simulink model "EvenorOddcheck"  (R2021a)
settings: Solver=FixedStepDiscrete  StartTime=0.0  StopTime=10.0  RelTol=1e-3
libraries: simulink x1
settings Model: Creator=Dell  LastModifiedBy=Dell
settings OptimizationCC: DefaultParameterBehavior=Inlined  EnhancedBackFolding=on  PassReuseOutputArgsAs=Individual arguments  ZeroExternalMemoryAtStartup=off  ZeroInternalMemoryAtStartup=off  OptimizeBlockOrder=speed  DifferentSizesBufferReuse=on  OptimizationCustomize=off  EfficientTunableParamExpr=on
settings DebuggingCC: ParameterTunabilityLossMsg=error
settings SFSimCC: MATLABDynamicMemAlloc=off
settings RTWCC: SystemTargetFile=ert.tlc  GenCodeOnly=on  TemplateMakefile=ert_default_tmf  GenerateReport=on  IncludeHyperlinkInReport=on  LaunchReport=on  GenerateTraceInfo=on
settings CodeAppCC: ForceParamTrailComments=on  IgnoreCustomStorageClasses=off  OperatorAnnotations=on  SimulinkDataObjDesc=on  SFDataObjDesc=on  InsertBlockDesc=on
settings ERTTargetCC: TargetLangStandard=C99 (ISO)  GenerateSampleERTMain=on  InlinedParameterPlacement=NonHierarchical  ERTCustomFileTemplate=example_file_process.tlc

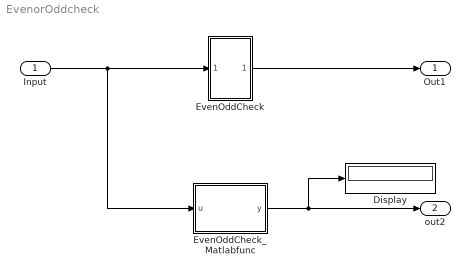
== system EvenorOddcheck ==
  Input : Inport  OutDataTypeStr=uint8
  Display : Display
  EvenOddCheck : Subsystem
  EvenOddCheck_Matlabfunc : MATLAB Function  TreatAsAtomicUnit=on
  Out1 : Outport  OutDataTypeStr=string
  out2 : Outport  Port=2
  wires:
  Input/1 -> EvenOddCheck_Matlabfunc/1(u), EvenOddCheck/1(In1)
  EvenOddCheck/1(Out1) -> Out1/1
  EvenOddCheck_Matlabfunc/1(y) -> Display/1, out2/1

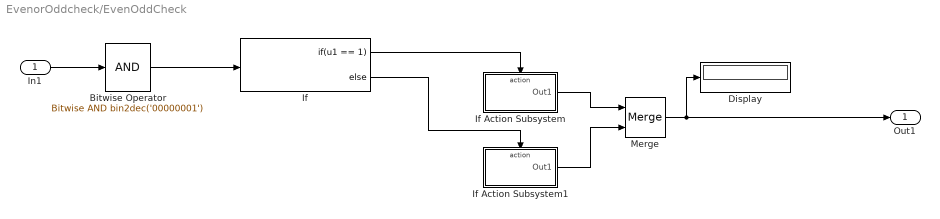
== system EvenorOddcheck/EvenOddCheck ==
  In1 : Inport
  Bitwise Operator : simulink/Logic and Bit Operations/Bitwise Operator  logicop=AND  UseBitMask=on  BitMask=bin2dec('00000001')  BitMaskRealWorld=Stored Integer
  Display : Display
  If : If  IfExpression=u1 == 1
  If Action Subsystem : Subsystem  TreatAsAtomicUnit=on
  If Action Subsystem1 : Subsystem  TreatAsAtomicUnit=on
  Merge : Merge
  Out1 : Outport
  wires:
  Bitwise Operator/1 -> If/1
  If Action Subsystem/1(Out1) -> Merge/1
  If Action Subsystem1/1(Out1) -> Merge/2
  In1/1 -> Bitwise Operator/1
  If/2 -> If Action Subsystem1/Action
  Merge/1 -> Out1/1, Display/1
  If/1 -> If Action Subsystem/Action

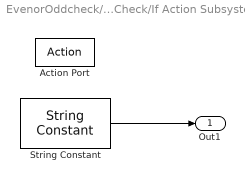
== system EvenorOddcheck/EvenOddCheck/If Action Subsystem ==
  Action Port : ActionPort  ActionPortLabel=if(u1 == 1)
  String Constant : StringConstant  String="\"Odd Number!\""
  Out1 : Outport  OutDataTypeStr=string
  wires:
  String Constant/1 -> Out1/1

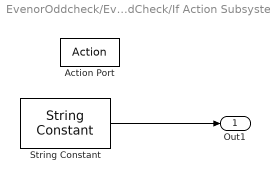
== system EvenorOddcheck/EvenOddCheck/If Action Subsystem1 ==
  Action Port : ActionPort  ActionPortLabel=else
  String Constant : StringConstant  String="\"Even Number!\""
  Out1 : Outport
  wires:
  String Constant/1 -> Out1/1

== matlab function EvenorOddcheck/EvenOddCheck_Matlabfunc ==
  data: u input; y output
function y = evenOddChecker(u)
    if mod(u, 2) == 0
        y = "even";
    else
        y = "odd";
    end
end
